simulink model "ledTrigger"  (R2016b)
settings: Solver=FixedStepDiscrete  StartTime=0.0  StopTime=10.0  RelTol=1e-3
settings Model: Creator=Radwa  LastModifiedBy=Radwa
settings SolverCC: EnableConcurrentExecution=on
settings DataIOCC: ReturnWorkspaceOutputs=on
settings OptimizationCC: DefaultParameterBehavior=Inlined  EnhancedBackFolding=on  PassReuseOutputArgsAs=Individual arguments
settings DebuggingCC: ParameterTunabilityLossMsg=error
settings SFSimCC: SimUseLocalCustomCode=on
settings RTWCC: SystemTargetFile=ert.tlc  GenCodeOnly=on  TemplateMakefile=ert_default_tmf  Description=Embedded Coder  GenerateReport=on  RTWUseLocalCustomCode=on  IncludeHyperlinkInReport=on  LaunchReport=on  GenerateTraceInfo=on  GenerateTraceReport=on  GenerateTraceReportSl=on  GenerateTraceReportSf=on  GenerateTraceReportEml=on
settings CodeAppCC: ForceParamTrailComments=on  IgnoreCustomStorageClasses=off  OperatorAnnotations=on  SimulinkDataObjDesc=on  SFDataObjDesc=on  InsertBlockDesc=on
settings ERTTargetCC: TargetLangStandard=C99 (ISO)  MultiwordLength=256  GenerateSampleERTMain=on  InlinedParameterPlacement=NonHierarchical  ERTCustomFileTemplate=example_file_process.tlc

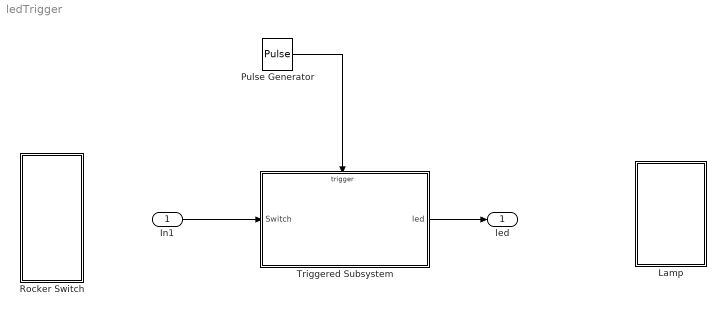
== system ledTrigger ==
  In1 : Inport
  Lamp : Subsystem  DialogController=hmiCreateDDGDialog  IsWebBlock=on  mask(MWDashboardBlock){webBlockId=57b8be76-9399-49d0-a523-996b8d4f9ea9, webBlockType=lamp, ShowInLibBrowser=on, ShowInitialText=on, HMISrcModelName=ledTrigger}
      mask prompts: webBlockType "WebBlock Type"; HMISrcModelName "Source Model"
      mask help: SimulinkHMI:dialogs:LampDialogDesc
      mask Help: helpview([docroot '/mapfiles/simulink.map'], 'hmi_lamp')
      mask Display:
      | if strcmp(get_param(bdroot(gcb),'BlockDiagramType'), 'library')
      |     image([(matlabroot) '/toolbox/simulink/hmi/icons/Lamp.png']);
      | end
  Pulse Generator : DiscretePulseGenerator  PulseType=Time based  Period=10  PulseWidth=5
  Rocker Switch : Subsystem  DialogController=hmiCreateDDGDialog  IsWebBlock=on  mask(MWDashboardBlock){webBlockId=09e56217-e9ad-4574-8c26-535ccc063de9, webBlockType=rockerswitch, ShowInLibBrowser=on, ShowInitialText=on, HMISrcModelName=ledTrigger}
      mask prompts: webBlockId "WebBlock Id"; webBlockType "WebBlock Type"; HMISrcModelName "Source Model"
      mask help: SimulinkHMI:dialogs:SwitchDialogDesc
      mask Help: helpview([docroot '/mapfiles/simulink.map'], 'hmi_rocker_switch')
      mask Display:
      | if strcmp(get_param(bdroot(gcb),'BlockDiagramType'), 'library')
      |     image([(matlabroot) '/toolbox/simulink/hmi/icons/RockerSwitch.png']);
      | end
  Triggered Subsystem : Subsystem  TreatAsAtomicUnit=on
  led : Outport
  wires:
  In1/1 -> Triggered Subsystem/1(Switch)
  Triggered Subsystem/1(led) -> led/1
  Pulse Generator/1 -> Triggered Subsystem/Trigger

== system ledTrigger/Lamp ==

== system ledTrigger/Rocker Switch ==

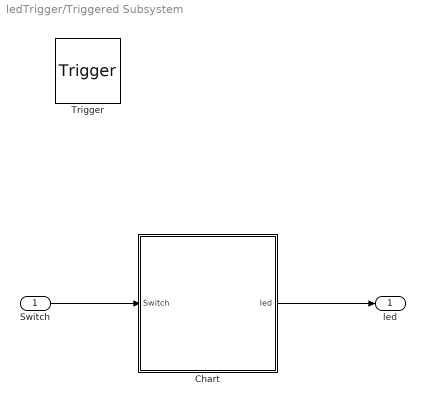
== system ledTrigger/Triggered Subsystem ==
  Switch : Inport
  Trigger : TriggerPort  VariantControl=Variant
  Chart : Stateflow chart  TreatAsAtomicUnit=on
  led : Outport
  wires:
  Switch/1 -> Chart/1(Switch)
  Chart/1(led) -> led/1

== stateflow chart ledTrigger/Triggered Subsystem/Chart ==
  (default) -> (junction 9) : %led_status
  (junction 9) -> (junction 10) [order 1] : [Switch==1]
  (junction 9) -> (junction 11) [order 2] : {led=0;}
  (junction 10) -> (junction 12) : {led=1;}
  (junction 12) -> (junction 11)
  (junction 11) -> (junction 13)
  data: led output =0; Switch input
